simulink model "minmax_task"  (Simulink 3.00)
libraries: logiclib x4, mathlib x3, analoglib x3, execlib x2, genlib x2, arclib x1

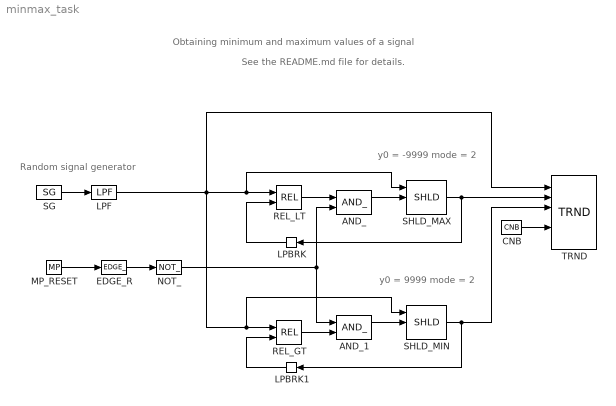
== system minmax_task ==
  note: y0 = 9999
      | mode = 2
  note: See the README.md file for details.
  note: Obtaining minimum and maximum values of a signal
  note: y0 = -9999
      | mode = 2
  note: Random signal
      | generator
  AND_ : logiclib/AND_
  AND_1 : logiclib/AND_
  CNB : mathlib/CNB  YCN=on
  EDGE_R : logiclib/EDGE_  iedge=1: Rising edge
  LPBRK : execlib/LPBRK  Orientation=left
  LPBRK1 : execlib/LPBRK  Orientation=left
  LPF : analoglib/LPF  fb=0.1  xi=0.707  ISSF=off
  MP_RESET : genlib/MP  pwidth=1  BSTATE=off  RPTF=off
  NOT_ : logiclib/NOT_
  REL_GT : mathlib/REL  irel=4: greater than (>)
  REL_LT : mathlib/REL  irel=3: less than (<)
  SG : genlib/SG  isig=4: RANDOM  amp=1  freq=1  phase=0  ifrunit=1: Hz  iphunit=1: degrees
  SHLD_MAX : analoglib/SHLD  y0=-9999  mode=2: Hold last value
  SHLD_MIN : analoglib/SHLD  y0=9999  mode=2: Hold last value
  TRND : arclib/TRND  n=3  l=1000  btype=8: Double  ptype1=1: Store  ptype2=1: Store  ptype3=1: Store  ptype4=1: Store  pfac=1  afac=0  arc=0  id=1  Title=Signal and its extremes
  wires:
  AND_/1 -> SHLD_MAX/2
  AND_1/1 -> SHLD_MIN/2
  CNB/1 -> TRND/5
  EDGE_R/1 -> NOT_/1
  LPBRK/1 -> REL_LT/2
  LPBRK1/1 -> REL_GT/2
  LPF/1 -> REL_LT/1, SHLD_MAX/1, TRND/1, REL_GT/1, SHLD_MIN/1
  MP_RESET/1 -> EDGE_R/1
  NOT_/1 -> AND_/2, AND_1/1
  REL_GT/1 -> AND_1/2
  REL_LT/1 -> AND_/1
  SG/1 -> LPF/1
  SHLD_MAX/1 -> LPBRK/1, TRND/2
  SHLD_MIN/1 -> LPBRK1/1, TRND/3
